simulink model "DigitalIO_block_demo"  (Simulink 8.1)
settings: Solver=FixedStepDiscrete  StartTime=0.0  StopTime=10.0  FixedStep=0.050  RelTol=1e-3
undefined symbols (not defined in the file or in its folder): A14, A7, B, B13, B7, B8, C5, D, L3, N3, P3, PD0, PD1, PD2, PD3, PD4, PD5, PD6, PD7, R10, R4
libraries: rappid_564xl_ec_toolbox x16
settings Model: Creator=r61406  LastModifiedBy=evarshavskaya
settings SolverCC: PositivePriorityOrder=on  AutoInsertRateTranBlk=on
settings DataIOCC: ExternalInput=off  InitialState=off  LimitDataPoints=off  SaveOutput=off  SignalLogging=off  SaveTime=off
settings OptimizationCC: InlineParams=on  EnableMemcpy=off  InitFltsAndDblsToZero=on  OptimizeModelRefInitCode=on  LifeSpan=1
settings DebuggingCC: InheritedTsInSrcMsg=none  SingleTaskRateTransMsg=error  UnconnectedInputMsg=error  UnconnectedOutputMsg=error  UnconnectedLineMsg=error  UnknownTsInhSupMsg=error  StrictBusMsg=Warning
settings HardwareCC: ProdLargestAtomicInteger=Long  ProdLargestAtomicFloat=Double  ProdIntDivRoundTo=Zero  ProdEndianess=BigEndian  ProdHWDeviceType=Freescale->32-bit PowerPC
settings RTWCC: SystemTargetFile=rappid564xl.tlc  MakeCommand=rappid_564xl_make_rtw  TemplateMakefile=rappid_564xl_default_tmf  PostCodeGenCommand=rappid_analyzegencode(buildInfo)  Description=RAppID Toolbox MPC564xL Code Generation Target (rappid)  ProcessScript=rappid564xl_make_rtw_hook
settings CodeAppCC: IgnoreCustomStorageClasses=off  CustomSymbolStrType=$N$R$M  InternalIdentifier=Classic
settings STFCustomTargetCC: CodeReplacementLibrary=ANSI_C  ModelReferenceCompliant=off  CombineOutputUpdateFcns=on  SuppressErrorStatus=on  ERTCustomFileBanners=on  SupportContinuousTime=off  SupportNonInlinedSFcns=off  MATLABClassNameForMDSCustomization=Simulink.SoftwareTarget.ERTCustomization  GRTInterface=off  SystemTargetFile=rappid564xl.tlc
settings ERTTargetCC: CodeReplacementLibrary=ANSI_C  MultiwordLength=2048  ModelReferenceCompliant=off  ParMdlRefBuildCompliant=off  CompOptLevelCompliant=off  ConcurrentExecutionCompliant=off  SuppressErrorStatus=on  ERTFirstTimeCompliant=off  ModelStepFunctionPrototypeControlCompliant=off  CPPClassGenCompliant=off  InlinedParameterPlacement=NonHierarchical  ERTCustomFileTemplate=example_file_process.tlc  ConvertIfToSwitch=off  SuppressUnreachableDefaultCases=off

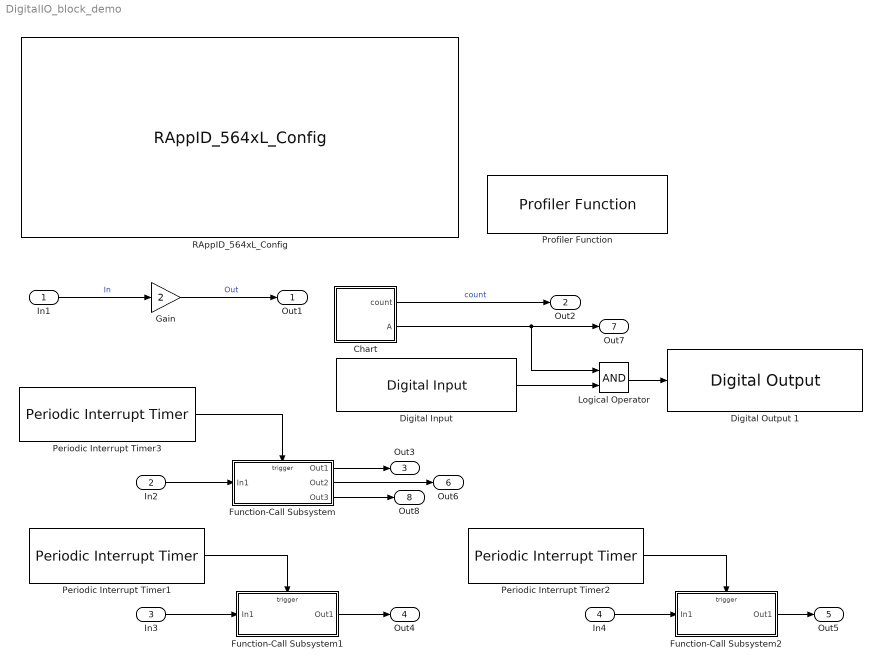
== system DigitalIO_block_demo ==
  In1 : Inport
  In2 : Inport  Port=2
  In3 : Inport  Port=3
  In4 : Inport  Port=4
  Chart : Stateflow chart  TreatAsAtomicUnit=on
  Digital Input : rappid_564xl_ec_toolbox/MPC564xL/General Purpose Blocks/Digital Input  gpio_outputs="51  : PD3  : [ 128 ] : [ A7 ]"  pinNum=[ 128 ]  pcrNum=51
  Digital Output 1 : rappid_564xl_ec_toolbox/MPC564xL/General Purpose Blocks/Digital Output   gpio_outputs="55  : PD7  : [ 37 ] : [ R4 ]"  pinNum=[ 37 ]  pcrNum=55
  Function-Call Subsystem : Subsystem  TreatAsAtomicUnit=on
      settings: RTWSystemCode=Nonreusable function
  Function-Call Subsystem1 : Subsystem  TreatAsAtomicUnit=on
      settings: RTWSystemCode=Nonreusable function
  Function-Call Subsystem2 : Subsystem  TreatAsAtomicUnit=on
      settings: RTWSystemCode=Nonreusable function
  Gain : Gain  Gain=2
  Logical Operator : Logic  AllPortsSameDT=off  OutDataTypeStr=boolean
  Periodic Interrupt Timer1 : rappid_564xl_ec_toolbox/MPC564xL/General Purpose Blocks/Periodic Interrupt Timer  pit_chan=2  pit_timeout=100  int_priority=12  pit_timeout_val=11999999
  Periodic Interrupt Timer2 : rappid_564xl_ec_toolbox/MPC564xL/General Purpose Blocks/Periodic Interrupt Timer  pit_chan=3  pit_timeout=250  int_priority=12  pit_timeout_val=29999999
  Periodic Interrupt Timer3 : rappid_564xl_ec_toolbox/MPC564xL/General Purpose Blocks/Periodic Interrupt Timer  pit_chan=1  pit_timeout=200  int_priority=12  pit_timeout_val=23999999
  "Profiler Function " : rappid_564xl_ec_toolbox/MPC564xL/Utility Blocks/Profiler Function   profile_indx=1
  RAppID_564xL_Config : rappid_564xl_ec_toolbox/MPC564xL/RAppID_564xL_Config  SystemClock=120  XTAL=40  MC_clock_60=12  MC_clock_80=16  MC_clock_120=10  SWG_clock_60=20  SWG_clock_80=13.334  SWG_clock_120=20  Compiler=CodeWarrior  MemTarget=RAM  Part=MPC5643L  Package=144 LQFP  global_int_priority=10  base_tick_priority=14  sys_task_supress=off  exception_handlers=off  stored_mdl_name=rappid_564xl_ec_toolbox  freemaster_interface=Oops  freemaster_rx_pin="LINFlex_0 Rx Pin 116 : \"PB[3]\""  freemaster_tx_pin="LINFlex_0 Tx Pin 114 : \"PB[2]\""  freemaster_interface_1=None  freemaster_enable=off  freemaster_rate=57600  freemaster_tx0_pin=18 : B[2] : 114 : A14  freemaster_rx0_pin=19 : B[3] : 116 : B13  freemaster_tx1_pin=57 : D[9] : 26 : L3  freemaster_rx1_pin=29 : B[13] : 60 : R10  freemaster_can_channel=1CH  freemater_can_speed=500K  freemaster_can_msgig=0x7AA  ccp_interface=None  ccp_enable=off  ccp_can_channel=CH1 (MB 0 - 1)  ccp_can_speed=500K  ccp_can_cro_id=256  ccp_can_dto_id=257  ccp_dev_id=RappID  ccp_dev_addr=0  ccp_odt=3  ccp_daq=3  pil_enable=off  pil_bam=on  comport=1  pil_rate=57600  bam_password_def=on  bam_password=0xFEEDFACECAFEBEEF  bam_sa_cs=off  bam_start_address=0x0  bam_code_size=0x7000  cons_dspi=on  cons_can=on  cons_adc=on  cons_pwm=on  cons_ctu=on  cons_swg=on  cons_eTimer=on  cons_fm=on
  Out1 : Outport
  Out2 : Outport  Port=2
  Out3 : Outport  Port=3
  Out4 : Outport  Port=4
  Out5 : Outport  Port=5
  Out6 : Outport  Port=6
  Out7 : Outport  Port=7
  Out8 : Outport  Port=8
  wires:
  In1/1 -> Gain/1  "In"
  Gain/1 -> Out1/1  "Out"
  Chart/1(count) -> Out2/1  "count"
  Function-Call Subsystem/1(Out1) -> Out3/1
  In2/1 -> Function-Call Subsystem/1(In1)
  Periodic Interrupt Timer3/1 -> Function-Call Subsystem/Trigger
  Function-Call Subsystem1/1(Out1) -> Out4/1
  In3/1 -> Function-Call Subsystem1/1(In1)
  Periodic Interrupt Timer1/1 -> Function-Call Subsystem1/Trigger
  Function-Call Subsystem2/1(Out1) -> Out5/1
  In4/1 -> Function-Call Subsystem2/1(In1)
  Periodic Interrupt Timer2/1 -> Function-Call Subsystem2/Trigger
  Chart/2(A) -> Out7/1, Logical Operator/1
  Function-Call Subsystem/2(Out2) -> Out6/1
  Function-Call Subsystem/3(Out3) -> Out8/1
  Logical Operator/1 -> Digital Output 1/1
  Digital Input/1 -> Logical Operator/2

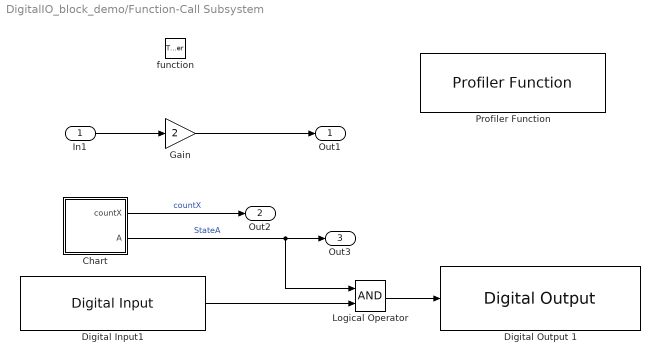
== system DigitalIO_block_demo/Function-Call Subsystem ==
  In1 : Inport
  function : TriggerPort  TriggerType=function-call
  Chart : Stateflow chart  TreatAsAtomicUnit=on
  Digital Input1 : rappid_564xl_ec_toolbox/MPC564xL/General Purpose Blocks/Digital Input  gpio_outputs="48  : PD0  : [ 125 ] : [ B8 ]"  pinNum=[ 125 ]  pcrNum=48
  Digital Output 1 : rappid_564xl_ec_toolbox/MPC564xL/General Purpose Blocks/Digital Output   gpio_outputs="52  : PD4  : [ 129 ] : [ B7 ]"  pinNum=[ 129 ]  pcrNum=52
  Gain : Gain  Gain=2
  Logical Operator : Logic  AllPortsSameDT=off  OutDataTypeStr=boolean
  "Profiler Function " : rappid_564xl_ec_toolbox/MPC564xL/Utility Blocks/Profiler Function   profile_indx=0
  Out1 : Outport
  Out2 : Outport  Port=2
  Out3 : Outport  Port=3
  wires:
  In1/1 -> Gain/1
  Gain/1 -> Out1/1
  Chart/1(countX) -> Out2/1  "countX"
  Chart/2(A) -> Out3/1, Logical Operator/1  "StateA"
  Digital Input1/1 -> Logical Operator/2
  Logical Operator/1 -> Digital Output 1/1

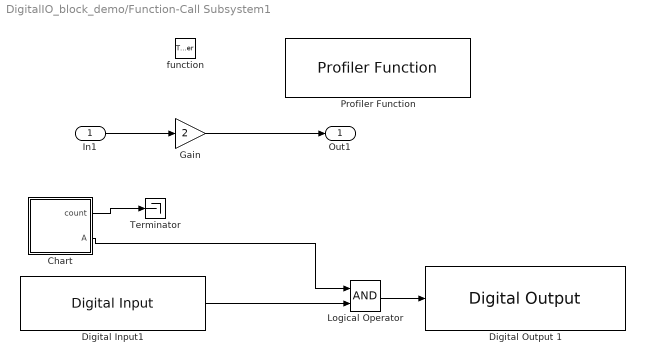
== system DigitalIO_block_demo/Function-Call Subsystem1 ==
  In1 : Inport
  function : TriggerPort  TriggerType=function-call
  Chart : Stateflow chart  TreatAsAtomicUnit=on
  Digital Input1 : rappid_564xl_ec_toolbox/MPC564xL/General Purpose Blocks/Digital Input  gpio_outputs="49  : PD1  : [ 3 ] : [ E3 ]"  pinNum=[ 3 ]  pcrNum=49
  Digital Output 1 : rappid_564xl_ec_toolbox/MPC564xL/General Purpose Blocks/Digital Output   gpio_outputs="53  : PD5  : [ 33 ] : [ N3 ]"  pinNum=[ 33 ]  pcrNum=53
  Gain : Gain  Gain=2
  Logical Operator : Logic  AllPortsSameDT=off  OutDataTypeStr=boolean
  "Profiler Function " : rappid_564xl_ec_toolbox/MPC564xL/Utility Blocks/Profiler Function   profile_indx=2
  Terminator : Terminator
  Out1 : Outport
  wires:
  Gain/1 -> Out1/1
  In1/1 -> Gain/1
  Chart/2(A) -> Logical Operator/1
  Chart/1(count) -> Terminator/1
  Digital Input1/1 -> Logical Operator/2
  Logical Operator/1 -> Digital Output 1/1

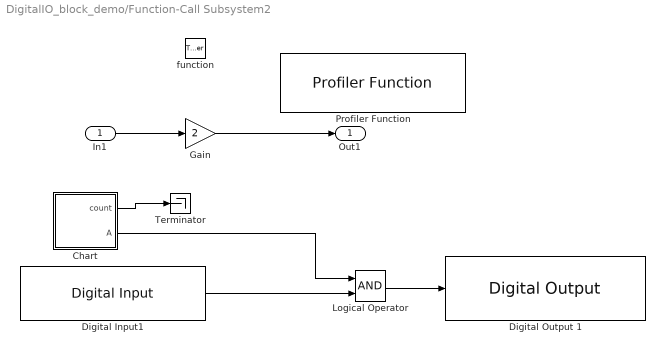
== system DigitalIO_block_demo/Function-Call Subsystem2 ==
  In1 : Inport
  function : TriggerPort  TriggerType=function-call
  Chart : Stateflow chart  TreatAsAtomicUnit=on
  Digital Input1 : rappid_564xl_ec_toolbox/MPC564xL/General Purpose Blocks/Digital Input  gpio_outputs="50  : PD2  : [ 140 ] : [ C5 ]"  pinNum=[ 140 ]  pcrNum=50
  Digital Output 1 : rappid_564xl_ec_toolbox/MPC564xL/General Purpose Blocks/Digital Output   gpio_outputs="54  : PD6  : [ 34 ] : [ P3 ]"  pinNum=[ 34 ]  pcrNum=54
  Gain : Gain  Gain=2
  Logical Operator : Logic  AllPortsSameDT=off  OutDataTypeStr=boolean
  "Profiler Function " : rappid_564xl_ec_toolbox/MPC564xL/Utility Blocks/Profiler Function   profile_indx=3
  Terminator : Terminator
  Out1 : Outport
  wires:
  In1/1 -> Gain/1
  Gain/1 -> Out1/1
  Chart/2(A) -> Logical Operator/1
  Chart/1(count) -> Terminator/1
  Digital Input1/1 -> Logical Operator/2
  Logical Operator/1 -> Digital Output 1/1

== stateflow chart Chart ==
  state A [parallel]
    settings: executionOrder=1
    state A
    state A1
    (default) -> A.A
    A.A -> A.A1
    A.A1 -> A.A : { count = count + 0.01;}
  state A1 [parallel]
    settings: executionOrder=2
    A1 -> (junction 10) : {a=0;}
    (junction 10) -> (junction 11) [order 1] : [a < 100]
        | {a=a+1;}
    (junction 10) -> (junction 11) [order 2] : {a=0;}
  data: count output double [0..10000]; A output boolean [0..1]; a local double [0..100]

== stateflow chart Function-Call Subsystem/Chart ==
  state A
  state A1
  (default) -> A
  A -> A1
  A1 -> A : { countX = countX + 0.01;}
  data: countX output single [0..10000]; A output boolean [0..1]

== stateflow chart Function-Call Subsystem1/Chart ==
  state A
  state A1
  (default) -> A : {count =0;}
  A -> A1
  A1 -> A : { count = count + 1;}
  data: count output double [0..10000]; A output boolean [0..1]

== stateflow chart Function-Call Subsystem2/Chart ==
  state A
  state A1
  (default) -> A
  A -> A1
  A1 -> A : { count = count + 0.01;}
  data: count output double [0..10000]; A output boolean [0..1]
